simulink subsystem "MPC8_nlpsol"  (R2022b)
settings: Solver=VariableStepAuto  StartTime=0.0  StopTime=10.0  RelTol=1e-3
undefined symbols (not defined in the file): param_global, param_MPC8, param_weight_init
settings Model: Creator=emu  LastModifiedBy=emu
settings OptimizationCC: ReuseModelBlockBuffer=on

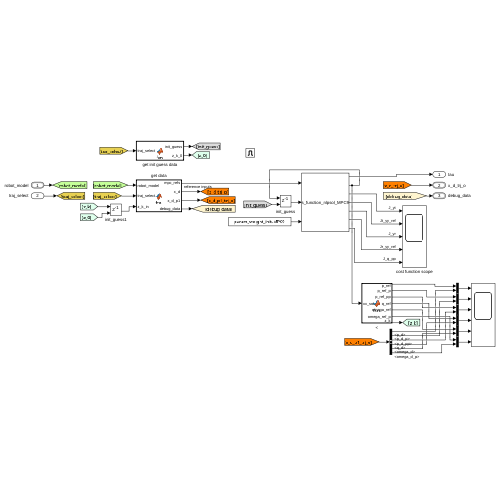
[thumbnail: Simulink's stored preview of the top-level diagram]
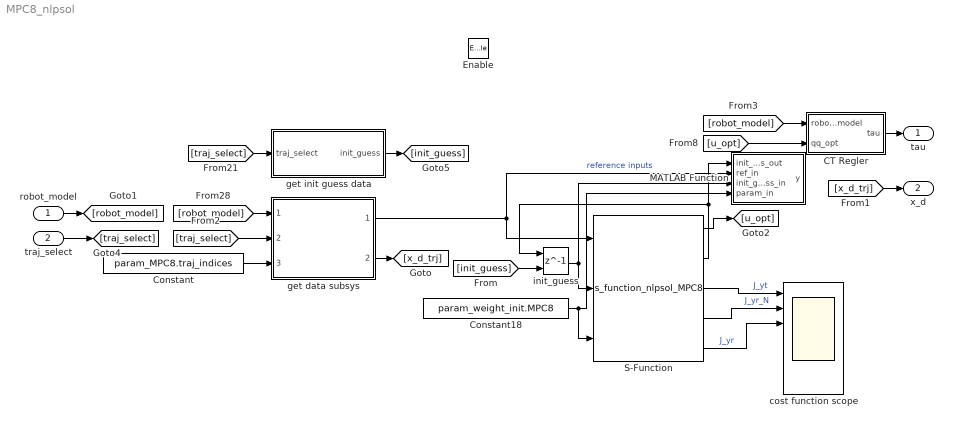
== system MPC8_nlpsol ==
  robot_model : Inport  OutDataTypeStr=Bus: robot_model
  traj_select : Inport  Port=2
  Enable : EnablePort
  CT Regler : MATLAB Function  TreatAsAtomicUnit=on
  Constant : Constant  Value=param_MPC8.traj_indices
  Constant18 : Constant  Value=param_weight_init.MPC8  VectorParams1D=off
  MATLAB Function : MATLAB Function  TreatAsAtomicUnit=on
  S-Function : S-Function  FunctionName=s_function_nlpsol_MPC8  Parameters='s_functions/fr3_no_hand_6dof/MPC8.casadi', 'MPC8'  SFunctionModules='MPC8'  SFunctionDeploymentMode=off  EnableBusSupport=off
  cost function scope : Scope  NumInputPorts=7
  get data subsys : Subsystem  ReferencedSubsystem=get_data_p_d_q_d_subsys
  get init guess data : MATLAB Function  TreatAsAtomicUnit=on
  init_guess : Delay  DelayLength=1  InitialConditionSource=Input port  InitialCondition=1  SampleTime=param_global.Ta
      settings: InputPortMap=u0,p4
  tau : Outport
  x_d : Outport  Port=2  OutDataTypeStr=Bus: x_d
  wires:
  S-Function/1 -> [u_opt]
  CT Regler/1(tau) -> tau/1
  S-Function/3 -> cost function scope/1  "J_yt"
  init_guess/1 -> S-Function/2, MATLAB Function/3(init_guess_in)
  S-Function/5 -> cost function scope/3  "J_yr"
  Constant18/1 -> S-Function/3, MATLAB Function/4(param_in)
  S-Function/2 -> init_guess/1, MATLAB Function/1(init_guess_out)
  S-Function/4 -> cost function scope/2  "J_yr_N"
  [u_opt] -> CT Regler/2(qq_opt)
  [robot_model] -> CT Regler/1(robot_model)
  traj_select/1 -> [traj_select]
  [traj_select] -> get data subsys/2
  [robot_model] -> get data subsys/1
  robot_model/1 -> [robot_model]
  get data subsys/1 -> MATLAB Function/2(ref_in), S-Function/1  "reference inputs"
  get init guess data/1(init_guess) -> [init_guess]
  [traj_select] -> get init guess data/1(traj_select)
  [init_guess] -> init_guess/2
  Constant/1 -> get data subsys/3
  get data subsys/2 -> [x_d_trj]
  [x_d_trj] -> x_d/1

== matlab function MPC8_nlpsol/CT Regler ==
  data: robot_model input Bus: robot_model; tau output; qq_opt input
function tau = fcn(robot_model, qq_opt)

if size(qq_opt, 2) ~= 0 && size(qq_opt, 1) ~= 1
    q_d_pp = qq_opt;

    M = robot_model.M;      % inertia matrix
    C_rnea = robot_model.C_rnea; % C_rnea(q, q_p) = C(q, q_p)q_p + g(q) = n(q, q_p)
    C = robot_model.C;
    g = robot_model.g;

    q = robot_model.q;
    q_p = robot_model.q_p;
    %tau = M*q_d_pp + C_rnea;

    %%{
    q_24_indices = [2 3]; % q2, q4 only (q3 ist deaktiviert daher ist q4 an index 3)

    M1 = M(q_24_indices, q_24_indices);

    tau1 = M1*q_d_pp;

    e = q - [0, -pi/4, -3 * pi/4, 0, pi/2, pi/4]';
    e_p = q_p;

    e(q_24_indices) = 0;
    e_p(q_24_indices) = 0;

    K_D_q = 3e1*eye(6);
    K_P_q = 3e1*eye(6);

    tau = M*(- K_D_q * e_p - K_P_q * e) + C * q_p + g; % Es soll kein CT Sondern ein PD Regler sein
    tau(q_24_indices) = tau(q_24_indices) + tau1;
    %}
else
    tau = zeros(6,1);
end

== matlab function MPC8_nlpsol/get init guess data ==
  data: traj_select input; param_MPC8_init_guess parameter; init_guess output
function init_guess   = fcn(traj_select, param_MPC8_init_guess)

%init_guess = param_MPC8_init_guess.init_guess(1,:);
init_guess = param_MPC8_init_guess.init_guess(traj_select,:);

== matlab function MPC8_nlpsol/MATLAB Function ==
  data: init_guess_out input; y output; ref_in input; init_guess_in input; param_in input
function y = fcn(init_guess_out, ref_in, init_guess_in, param_in)

y = 0;
